simulink model "qint_plant"  (Simulink 7.5)
settings: Solver=ode8  StartTime=0.0  StopTime=inf  FixedStep=0.002  RelTol=1e-3
undefined symbols (not defined in the file): passive_control, SectorSearch, serial
libraries: instrumentlib x3
settings Model: Creator=jporter  LastModifiedBy=jporter  BufferReuse=off
settings SolverCC: AutoInsertRateTranBlk=on
settings DataIOCC: LimitDataPoints=off  SaveOutput=off  SignalLogging=off  SaveTime=off
settings OptimizationCC: BlockReduction=off  OptimizeBlockIOStorage=off  BufferReuse=off  ExpressionFolding=off  LocalBlockOutputs=off  InitFltsAndDblsToZero=on
settings DebuggingCC: StrictBusMsg=Warning
settings HardwareCC: ProdIntDivRoundTo=Zero  ProdEndianess=LittleEndian  ProdHWDeviceType=Generic->32-bit x86 compatible  TargetEndianess=LittleEndian  TargetHWDeviceType=MATLAB Host  ProdEqTarget=off
settings RTWCC: SystemTargetFile=rsim.tlc  TemplateMakefile=rsim_default_tmf  Description=Rapid Simulation Target  GenerateReport=on  ProcessScript=rsim_make_rtw_hook  LaunchReport=on  RTWCompilerOptimization=On
settings RSimTargetCC: TargetFunctionLibrary=ANSI_C  ERTMultiwordTypeDef=System defined  ERTCodeCoverageTool=None  ERTMultiwordLength=256  IsPILTarget=off  EnableShiftOperators=on  PortableWordSizes=off

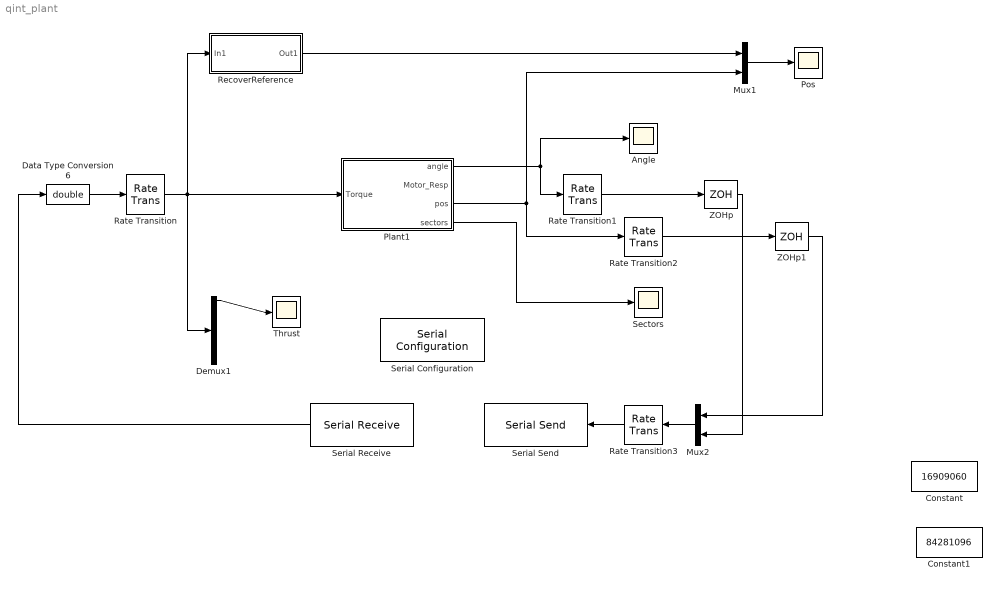
== system qint_plant ==
  Angle : Scope
      settings: SaveName=AngleData  MaxDataPoints=500000
  Constant : Constant  Value=16909060  OutDataTypeMode=uint32  OutDataType=sfix(16)  OutScaling=2^0  OutDataTypeStr=uint32  SampleTime=0.02
  Constant1 : Constant  Value=84281096  OutDataTypeMode=uint32  OutDataType=sfix(16)  OutScaling=2^0  OutDataTypeStr=uint32  SampleTime=0.02
  Data Type Conversion6 : DataTypeConversion  OutDataTypeMode=double  OutDataType=sfix(16)  OutScaling=2^0  OutDataTypeStr=double
  Demux1 : Demux  Outputs=9
  Mux1 : Mux  Inputs=2
  Mux2 : Mux  Inputs=2
  Plant1 : Subsystem
  Pos : Scope
      settings: SaveName=PosData  MaxDataPoints=500000
  Rate Transition : RateTransition  Deterministic=off
  Rate Transition1 : RateTransition  Deterministic=off  OutPortSampleTimeOpt=Inherit  OutPortSampleTimeMultiple=2
  Rate Transition2 : RateTransition  Deterministic=off  OutPortSampleTimeOpt=Inherit  OutPortSampleTimeMultiple=2
  Rate Transition3 : RateTransition  Deterministic=off  OutPortSampleTimeOpt=Inherit  OutPortSampleTimeMultiple=2
  RecoverReference : Subsystem
  Sectors : Scope
      settings: SaveName=SectorData  MaxDataPoints=500000
  Serial Configuration : instrumentlib/Serial Configuration  Priority=-200000  DialogController=instrumentcreatedialog  DialogControllerArgs=DataTag0  ComPortMenu=/dev/ttyUSB0  ComPort=/dev/ttyUSB0  ObjConstructor=serial('/dev/ttyUSB0');  BaudRate=57600  DataBits=8  Parity=none  StopBits=1  FlowControl=none  Timeout=0.05  ByteOrder=LittleEndian
  Serial Receive : instrumentlib/Serial Receive  DialogController=instrumentcreatedialog  DialogControllerArgs=DataTag1  ComPortMenu=/dev/ttyUSB0  ComPort=/dev/ttyUSB0  ObjConstructor=serial('/dev/ttyUSB0');  Header=char([147])  Terminator=<none>  DataSize="[9  1]"  DataType=single  EnableBlockingMode=on  ActionDataUnavailable=Output last received value  CustomValue=0  SampleTime=0.02
  Serial Send : instrumentlib/Serial Send  DialogController=instrumentcreatedialog  DialogControllerArgs=DataTag2  ComPortMenu=/dev/ttyUSB0  ComPort=/dev/ttyUSB0  ObjConstructor=serial('/dev/ttyUSB0');  Header=char([147])  Terminator=<none>  EnableBlockingMode=on
  Thrust : Scope
      settings: SaveName=ThrustData  MaxDataPoints=500000
  ZOHp : ZeroOrderHold  SampleTime=0.02
  ZOHp1 : ZeroOrderHold  SampleTime=0.02
  wires:
  Rate Transition1/1 -> ZOHp/1
  Data Type Conversion6/1 -> Rate Transition/1
  Plant1/1(angle) -> Rate Transition1/1, Angle/1
  Rate Transition2/1 -> ZOHp1/1
  Mux2/1 -> Rate Transition3/1
  ZOHp1/1 -> Mux2/1
  ZOHp/1 -> Mux2/2
  Plant1/3(pos) -> Mux1/2, Rate Transition2/1
  Rate Transition/1 -> Plant1/1(Torque), Demux1/1, RecoverReference/1(In1)
  RecoverReference/1(Out1) -> Mux1/1
  Mux1/1 -> Pos/1
  Serial Receive/1 -> Data Type Conversion6/1
  Demux1/1 -> Thrust/1
  Plant1/4(sectors) -> Sectors/1
  Rate Transition3/1 -> Serial Send/1

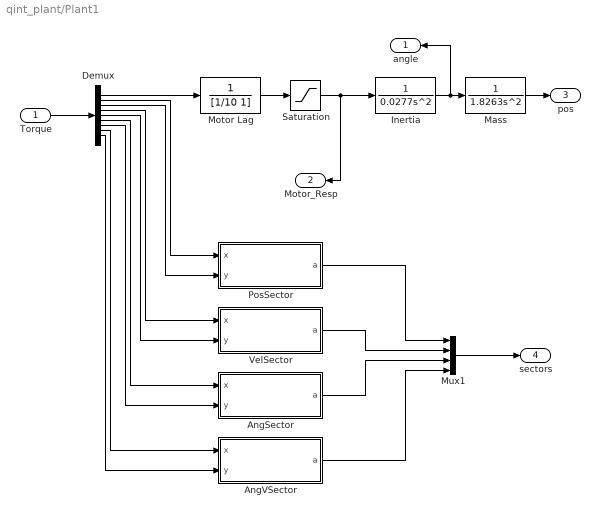
== system qint_plant/Plant1 ==
  Torque : Inport
  AngSector : Subsystem  AncestorBlock=passive_control/SectorSearch
  AngVSector : Subsystem  AncestorBlock=passive_control/SectorSearch
  Demux : Demux  Outputs=9
  Inertia : TransferFcn  Denominator=[0.0277 0 0]
  Mass : TransferFcn  Denominator=[1.8263 0 0]
  Motor Lag : TransferFcn  Denominator=[1/10 1]
  Mux1 : Mux
  PosSector : Subsystem  AncestorBlock=passive_control/SectorSearch
  Saturation : Saturate  UpperLimit=40  LowerLimit=-40  OutDataType=sfix(16)  OutScaling=2^0
  VelSector : Subsystem  AncestorBlock=passive_control/SectorSearch
  angle : Outport
  Motor_Resp : Outport  Port=2
  pos : Outport  Port=3
  sectors : Outport  Port=4
  wires:
  Motor Lag/1 -> Saturation/1
  Saturation/1 -> Inertia/1, Motor_Resp/1
  Inertia/1 -> Mass/1, angle/1
  Mass/1 -> pos/1
  Torque/1 -> Demux/1
  Demux/1 -> Motor Lag/1
  Demux/2 -> PosSector/1(x)
  Demux/3 -> PosSector/2(y)
  Demux/4 -> VelSector/1(x)
  Demux/5 -> VelSector/2(y)
  Demux/6 -> AngSector/1(x)
  Demux/7 -> AngSector/2(y)
  Demux/8 -> AngVSector/1(x)
  Demux/9 -> AngVSector/2(y)
  PosSector/1(a) -> Mux1/1
  VelSector/1(a) -> Mux1/2
  AngSector/1(a) -> Mux1/3
  AngVSector/1(a) -> Mux1/4
  Mux1/1 -> sectors/1

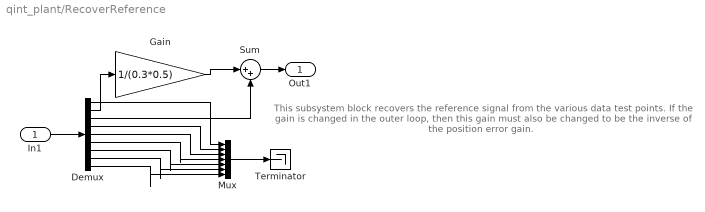
== system qint_plant/RecoverReference ==
  note: This subsystem block recovers the
      | reference signal from the various data
      | test points.  If the gain is changed in the
      | outer loop, then this gain must also be
      | changed to be the inverse of the position
      | error gain.
  In1 : Inport
  Demux : Demux  Outputs=9
  Gain : Gain  Gain=1/(0.3*0.5)  ParameterDataType=fixdt(1, 16)  ParameterScaling=2^0  OutDataType=fixdt(1, 16)  OutScaling=2^0
  Mux : Mux  Inputs=7
  Sum : Sum  Inputs=|++  OutDataType=fixdt(1, 16)  OutScaling=2^0
  Terminator : Terminator
  Out1 : Outport
  wires:
  Demux/2 -> Gain/1
  Gain/1 -> Sum/1
  Demux/3 -> Sum/2
  In1/1 -> Demux/1
  Sum/1 -> Out1/1
  Demux/1 -> Mux/1
  Demux/4 -> Mux/2
  Demux/5 -> Mux/3
  Demux/6 -> Mux/4
  Demux/7 -> Mux/5
  Demux/8 -> Mux/6
  Demux/9 -> Mux/7
  Mux/1 -> Terminator/1

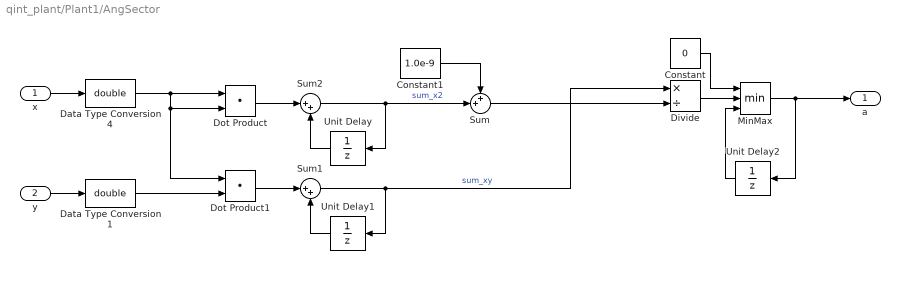
== system qint_plant/Plant1/AngSector ==
  x : Inport  OutDataType=sfix(16)  OutScaling=2^0
  y : Inport  Port=2  OutDataType=sfix(16)  OutScaling=2^0
  Constant : Constant  Value=0  OutDataTypeMode=double  OutDataType=sfix(16)  OutScaling=2^0  OutDataTypeStr=double
  Constant1 : Constant  Value=1.0e-9  OutDataTypeMode=double  OutDataType=sfix(16)  OutScaling=2^0  OutDataTypeStr=double
  Data Type Conversion1 : DataTypeConversion  OutDataTypeMode=double  OutDataType=sfix(16)  OutScaling=2^0  OutDataTypeStr=double
  Data Type Conversion4 : DataTypeConversion  OutDataTypeMode=double  OutDataType=sfix(16)  OutScaling=2^0  OutDataTypeStr=double
  Divide : Product  Inputs=*/  OutDataType=sfix(16)  OutScaling=2^-10
  Dot Product : DotProduct  OutDataType=sfix(16)  OutScaling=2^-10  InputSameDT=on  OutDataTypeStr=Inherit: Inherit via internal rule
  Dot Product1 : DotProduct  OutDataType=sfix(16)  OutScaling=2^-10  InputSameDT=on  OutDataTypeStr=Inherit: Inherit via internal rule
  MinMax : MinMax  Inputs=3  OutDataTypeMode=double  OutDataType=sfix(16)  OutScaling=2^0  OutDataTypeStr=double
  Sum : Sum  Inputs=++|  OutDataType=sfix(16)  OutScaling=2^0
  Sum1 : Sum  Inputs=|++  OutDataType=sfix(16)  OutScaling=2^0
  Sum2 : Sum  Inputs=|++  OutDataType=sfix(16)  OutScaling=2^0
  Unit Delay : UnitDelay  SampleTime=-1
  Unit Delay1 : UnitDelay  SampleTime=-1
  Unit Delay2 : UnitDelay  SampleTime=-1
  a : Outport  OutDataType=sfix(16)  OutScaling=2^0
  wires:
  Constant1/1 -> Sum/1
  Sum/1 -> Divide/2
  Unit Delay2/1 -> MinMax/3
  Divide/1 -> MinMax/2
  Constant/1 -> MinMax/1
  MinMax/1 -> Unit Delay2/1, a/1
  y/1 -> Data Type Conversion1/1
  x/1 -> Data Type Conversion4/1
  Dot Product1/1 -> Sum1/1
  Unit Delay1/1 -> Sum1/2
  Sum1/1 -> Divide/1, Unit Delay1/1  "sum_xy"
  Dot Product/1 -> Sum2/1
  Unit Delay/1 -> Sum2/2
  Sum2/1 -> Sum/2, Unit Delay/1  "sum_x2"
  Data Type Conversion4/1 -> Dot Product1/1, Dot Product/2, Dot Product/1
  Data Type Conversion1/1 -> Dot Product1/2

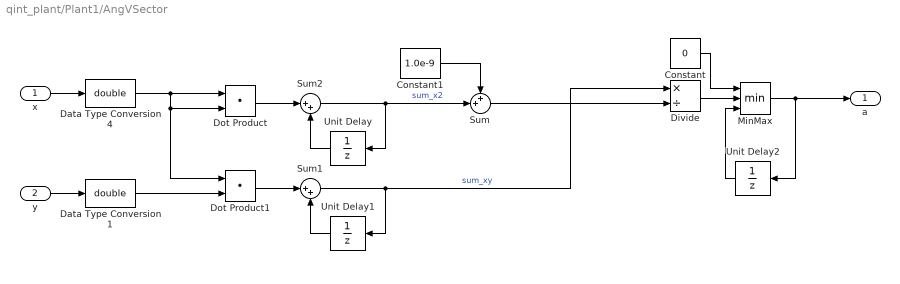
== system qint_plant/Plant1/AngVSector ==
  x : Inport  OutDataType=sfix(16)  OutScaling=2^0
  y : Inport  Port=2  OutDataType=sfix(16)  OutScaling=2^0
  Constant : Constant  Value=0  OutDataTypeMode=double  OutDataType=sfix(16)  OutScaling=2^0  OutDataTypeStr=double
  Constant1 : Constant  Value=1.0e-9  OutDataTypeMode=double  OutDataType=sfix(16)  OutScaling=2^0  OutDataTypeStr=double
  Data Type Conversion1 : DataTypeConversion  OutDataTypeMode=double  OutDataType=sfix(16)  OutScaling=2^0  OutDataTypeStr=double
  Data Type Conversion4 : DataTypeConversion  OutDataTypeMode=double  OutDataType=sfix(16)  OutScaling=2^0  OutDataTypeStr=double
  Divide : Product  Inputs=*/  OutDataType=sfix(16)  OutScaling=2^-10
  Dot Product : DotProduct  OutDataType=sfix(16)  OutScaling=2^-10  InputSameDT=on  OutDataTypeStr=Inherit: Inherit via internal rule
  Dot Product1 : DotProduct  OutDataType=sfix(16)  OutScaling=2^-10  InputSameDT=on  OutDataTypeStr=Inherit: Inherit via internal rule
  MinMax : MinMax  Inputs=3  OutDataTypeMode=double  OutDataType=sfix(16)  OutScaling=2^0  OutDataTypeStr=double
  Sum : Sum  Inputs=++|  OutDataType=sfix(16)  OutScaling=2^0
  Sum1 : Sum  Inputs=|++  OutDataType=sfix(16)  OutScaling=2^0
  Sum2 : Sum  Inputs=|++  OutDataType=sfix(16)  OutScaling=2^0
  Unit Delay : UnitDelay  SampleTime=-1
  Unit Delay1 : UnitDelay  SampleTime=-1
  Unit Delay2 : UnitDelay  SampleTime=-1
  a : Outport  OutDataType=sfix(16)  OutScaling=2^0
  wires:
  Constant1/1 -> Sum/1
  Sum/1 -> Divide/2
  Unit Delay2/1 -> MinMax/3
  Divide/1 -> MinMax/2
  Constant/1 -> MinMax/1
  MinMax/1 -> Unit Delay2/1, a/1
  y/1 -> Data Type Conversion1/1
  x/1 -> Data Type Conversion4/1
  Dot Product1/1 -> Sum1/1
  Unit Delay1/1 -> Sum1/2
  Sum1/1 -> Divide/1, Unit Delay1/1  "sum_xy"
  Dot Product/1 -> Sum2/1
  Unit Delay/1 -> Sum2/2
  Sum2/1 -> Sum/2, Unit Delay/1  "sum_x2"
  Data Type Conversion4/1 -> Dot Product1/1, Dot Product/2, Dot Product/1
  Data Type Conversion1/1 -> Dot Product1/2

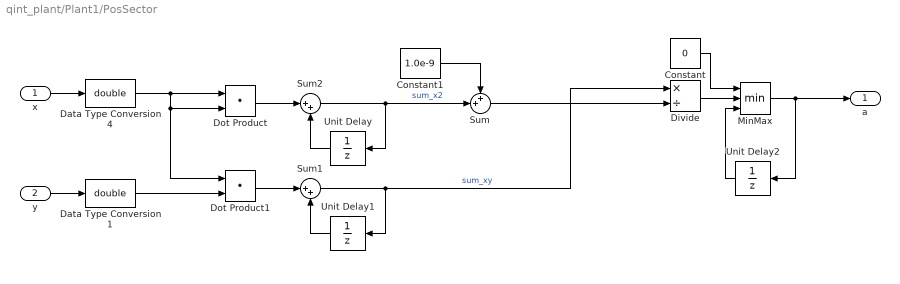
== system qint_plant/Plant1/PosSector ==
  x : Inport  OutDataType=sfix(16)  OutScaling=2^0
  y : Inport  Port=2  OutDataType=sfix(16)  OutScaling=2^0
  Constant : Constant  Value=0  OutDataTypeMode=double  OutDataType=sfix(16)  OutScaling=2^0  OutDataTypeStr=double
  Constant1 : Constant  Value=1.0e-9  OutDataTypeMode=double  OutDataType=sfix(16)  OutScaling=2^0  OutDataTypeStr=double
  Data Type Conversion1 : DataTypeConversion  OutDataTypeMode=double  OutDataType=sfix(16)  OutScaling=2^0  OutDataTypeStr=double
  Data Type Conversion4 : DataTypeConversion  OutDataTypeMode=double  OutDataType=sfix(16)  OutScaling=2^0  OutDataTypeStr=double
  Divide : Product  Inputs=*/  OutDataType=sfix(16)  OutScaling=2^-10
  Dot Product : DotProduct  OutDataType=sfix(16)  OutScaling=2^-10  InputSameDT=on  OutDataTypeStr=Inherit: Inherit via internal rule
  Dot Product1 : DotProduct  OutDataType=sfix(16)  OutScaling=2^-10  InputSameDT=on  OutDataTypeStr=Inherit: Inherit via internal rule
  MinMax : MinMax  Inputs=3  OutDataTypeMode=double  OutDataType=sfix(16)  OutScaling=2^0  OutDataTypeStr=double
  Sum : Sum  Inputs=++|  OutDataType=sfix(16)  OutScaling=2^0
  Sum1 : Sum  Inputs=|++  OutDataType=sfix(16)  OutScaling=2^0
  Sum2 : Sum  Inputs=|++  OutDataType=sfix(16)  OutScaling=2^0
  Unit Delay : UnitDelay  SampleTime=-1
  Unit Delay1 : UnitDelay  SampleTime=-1
  Unit Delay2 : UnitDelay  SampleTime=-1
  a : Outport  OutDataType=sfix(16)  OutScaling=2^0
  wires:
  Constant1/1 -> Sum/1
  Sum/1 -> Divide/2
  Unit Delay2/1 -> MinMax/3
  Divide/1 -> MinMax/2
  Constant/1 -> MinMax/1
  MinMax/1 -> Unit Delay2/1, a/1
  y/1 -> Data Type Conversion1/1
  x/1 -> Data Type Conversion4/1
  Dot Product1/1 -> Sum1/1
  Unit Delay1/1 -> Sum1/2
  Sum1/1 -> Divide/1, Unit Delay1/1  "sum_xy"
  Dot Product/1 -> Sum2/1
  Unit Delay/1 -> Sum2/2
  Sum2/1 -> Sum/2, Unit Delay/1  "sum_x2"
  Data Type Conversion4/1 -> Dot Product1/1, Dot Product/2, Dot Product/1
  Data Type Conversion1/1 -> Dot Product1/2

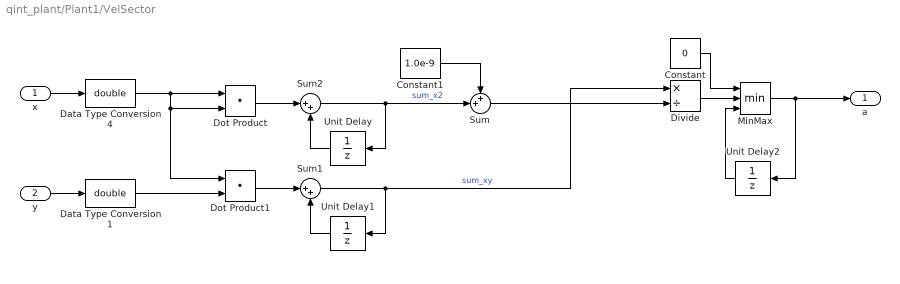
== system qint_plant/Plant1/VelSector ==
  x : Inport  OutDataType=sfix(16)  OutScaling=2^0
  y : Inport  Port=2  OutDataType=sfix(16)  OutScaling=2^0
  Constant : Constant  Value=0  OutDataTypeMode=double  OutDataType=sfix(16)  OutScaling=2^0  OutDataTypeStr=double
  Constant1 : Constant  Value=1.0e-9  OutDataTypeMode=double  OutDataType=sfix(16)  OutScaling=2^0  OutDataTypeStr=double
  Data Type Conversion1 : DataTypeConversion  OutDataTypeMode=double  OutDataType=sfix(16)  OutScaling=2^0  OutDataTypeStr=double
  Data Type Conversion4 : DataTypeConversion  OutDataTypeMode=double  OutDataType=sfix(16)  OutScaling=2^0  OutDataTypeStr=double
  Divide : Product  Inputs=*/  OutDataType=sfix(16)  OutScaling=2^-10
  Dot Product : DotProduct  OutDataType=sfix(16)  OutScaling=2^-10  InputSameDT=on  OutDataTypeStr=Inherit: Inherit via internal rule
  Dot Product1 : DotProduct  OutDataType=sfix(16)  OutScaling=2^-10  InputSameDT=on  OutDataTypeStr=Inherit: Inherit via internal rule
  MinMax : MinMax  Inputs=3  OutDataTypeMode=double  OutDataType=sfix(16)  OutScaling=2^0  OutDataTypeStr=double
  Sum : Sum  Inputs=++|  OutDataType=sfix(16)  OutScaling=2^0
  Sum1 : Sum  Inputs=|++  OutDataType=sfix(16)  OutScaling=2^0
  Sum2 : Sum  Inputs=|++  OutDataType=sfix(16)  OutScaling=2^0
  Unit Delay : UnitDelay  SampleTime=-1
  Unit Delay1 : UnitDelay  SampleTime=-1
  Unit Delay2 : UnitDelay  SampleTime=-1
  a : Outport  OutDataType=sfix(16)  OutScaling=2^0
  wires:
  Constant1/1 -> Sum/1
  Sum/1 -> Divide/2
  Unit Delay2/1 -> MinMax/3
  Divide/1 -> MinMax/2
  Constant/1 -> MinMax/1
  MinMax/1 -> Unit Delay2/1, a/1
  y/1 -> Data Type Conversion1/1
  x/1 -> Data Type Conversion4/1
  Dot Product1/1 -> Sum1/1
  Unit Delay1/1 -> Sum1/2
  Sum1/1 -> Divide/1, Unit Delay1/1  "sum_xy"
  Dot Product/1 -> Sum2/1
  Unit Delay/1 -> Sum2/2
  Sum2/1 -> Sum/2, Unit Delay/1  "sum_x2"
  Data Type Conversion4/1 -> Dot Product1/1, Dot Product/2, Dot Product/1
  Data Type Conversion1/1 -> Dot Product1/2
